simulink model "linear_pto_example"  (R2014a)
settings: Solver=ode45  StartTime=0.0  StopTime=10.0  RelTol=1e-3
undefined symbols (not defined in the file or in its folder): A_bore, A_rod, body, Gen_Damp, hyd_mot_eff, Jtot, p_hp, pto, V_hp, V_tot, Vg
libraries: WECSim_Lib x3
settings Model: Creator=kmruehl  LastModifiedBy=kmruehl
settings DebuggingCC: UnderspecifiedInitializationDetection=Classic  StateNameClashWarn=warning

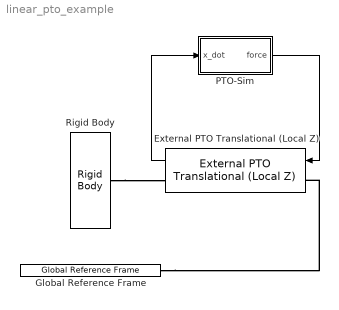
== system linear_pto_example ==
  External PTO Translational (Local Z) : WECSim_Lib/PTOs/External PTO  Translational (Local Z)  pto=pto(1)
      settings: AttributesFormatString=%<pto>
  Global Reference Frame : WECSim_Lib/Frames/Global Reference Frame  waves=waves  simu=simu
  PTO-Sim : Subsystem
  Rigid Body : WECSim_Lib/Body Elements/Rigid Body  Coupling=No  body=body(1)
      settings: AttributesFormatString=%<body>
  wires:
  External PTO Translational (Local Z)/1 -> PTO-Sim/1(x_dot)
  PTO-Sim/1(force) -> External PTO Translational (Local Z)/1
  connections:
  Rigid Body/RConn1 -- External PTO Translational (Local Z)/RConn1
  Global Reference Frame/RConn1 -- External PTO Translational (Local Z)/LConn1

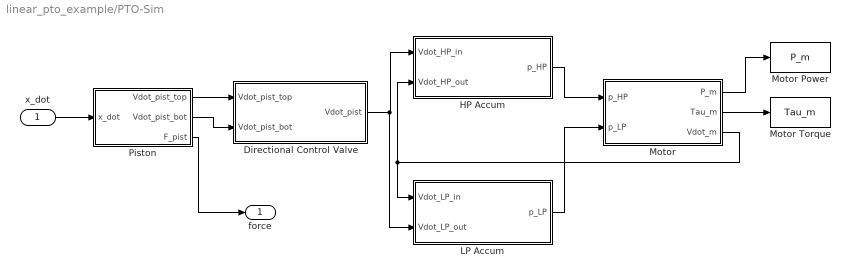
== system linear_pto_example/PTO-Sim ==
  x_dot : Inport
  Directional Control Valve : Subsystem
  HP Accum : Subsystem
  LP Accum : Subsystem
  Motor : Subsystem
  Motor Power : ToWorkspace  VariableName=P_m  SaveFormat=Timeseries  SampleTime=-1
  Motor Torque : ToWorkspace  VariableName=Tau_m  SaveFormat=Timeseries  SampleTime=-1
  Piston : Subsystem
  force : Outport
  wires:
  x_dot/1 -> Piston/1(x_dot)
  Motor/1(P_m) -> Motor Power/1
  Motor/2(Tau_m) -> Motor Torque/1
  Piston/2(Vdot_pist_bot) -> Directional Control Valve/2(Vdot_pist_bot)
  Piston/1(Vdot_pist_top) -> Directional Control Valve/1(Vdot_pist_top)
  Directional Control Valve/1(Vdot_pist) -> LP Accum/2(Vdot_LP_out), HP Accum/1(Vdot_HP_in)
  HP Accum/1(p_HP) -> Motor/1(p_HP)
  LP Accum/1(p_LP) -> Motor/2(p_LP)
  Motor/3(Vdot_m) -> LP Accum/1(Vdot_LP_in), HP Accum/2(Vdot_HP_out)
  Piston/3(F_pist) -> force/1

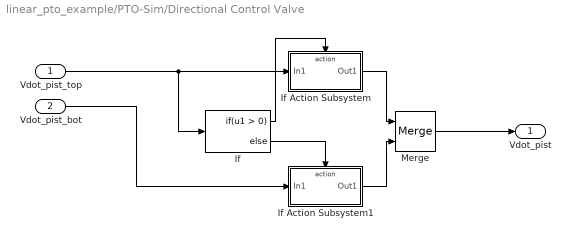
== system linear_pto_example/PTO-Sim/Directional Control Valve ==
  Vdot_pist_top : Inport
  Vdot_pist_bot : Inport  Port=2
  If : If
  If Action Subsystem : Subsystem  TreatAsAtomicUnit=on
  If Action Subsystem1 : Subsystem  TreatAsAtomicUnit=on
  Merge : Merge
  Vdot_pist : Outport
  wires:
  Vdot_pist_top/1 -> If/1, If Action Subsystem/1(In1)
  If/1 -> If Action Subsystem/Action
  If/2 -> If Action Subsystem1/Action
  If Action Subsystem/1(Out1) -> Merge/1
  If Action Subsystem1/1(Out1) -> Merge/2
  Vdot_pist_bot/1 -> If Action Subsystem1/1(In1)
  Merge/1 -> Vdot_pist/1

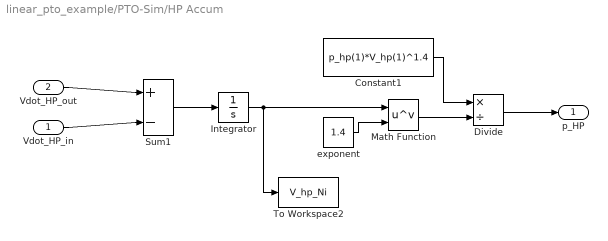
== system linear_pto_example/PTO-Sim/HP Accum ==
  Vdot_HP_in : Inport
  Vdot_HP_out : Inport  Port=2
  Constant1 : Constant  Value=p_hp(1)*V_hp(1)^1.4
  Divide : Product  Inputs=*/
  Integrator : Integrator  InitialCondition=V_hp(1)
  Math Function : Math  Operator=pow  SaturateOnIntegerOverflow=on
  Sum1 : Sum  Inputs=+|-
  To Workspace2 : ToWorkspace  VariableName=V_hp_Ni  SampleTime=-1
  exponent : Constant  Value=1.4
  p_HP : Outport
  wires:
  Integrator/1 -> Math Function/1, To Workspace2/1
  Divide/1 -> p_HP/1
  Math Function/1 -> Divide/2
  exponent/1 -> Math Function/2
  Constant1/1 -> Divide/1
  Sum1/1 -> Integrator/1
  Vdot_HP_in/1 -> Sum1/2
  Vdot_HP_out/1 -> Sum1/1

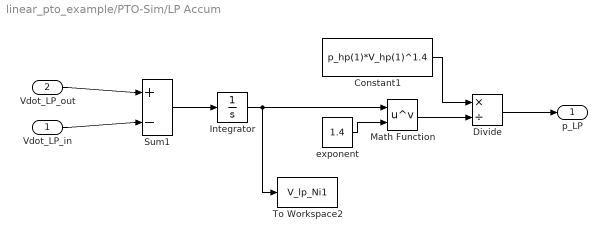
== system linear_pto_example/PTO-Sim/LP Accum ==
  Vdot_LP_in : Inport
  Vdot_LP_out : Inport  Port=2
  Constant1 : Constant  Value=p_hp(1)*V_hp(1)^1.4
  Divide : Product  Inputs=*/
  Integrator : Integrator  InitialCondition=V_hp(1)
  Math Function : Math  Operator=pow  SaturateOnIntegerOverflow=on
  Sum1 : Sum  Inputs=+|-
  To Workspace2 : ToWorkspace  VariableName=V_lp_Ni1  SampleTime=-1
  exponent : Constant  Value=1.4
  p_LP : Outport
  wires:
  Integrator/1 -> Math Function/1, To Workspace2/1
  Divide/1 -> p_LP/1
  Math Function/1 -> Divide/2
  exponent/1 -> Math Function/2
  Constant1/1 -> Divide/1
  Sum1/1 -> Integrator/1
  Vdot_LP_in/1 -> Sum1/2
  Vdot_LP_out/1 -> Sum1/1

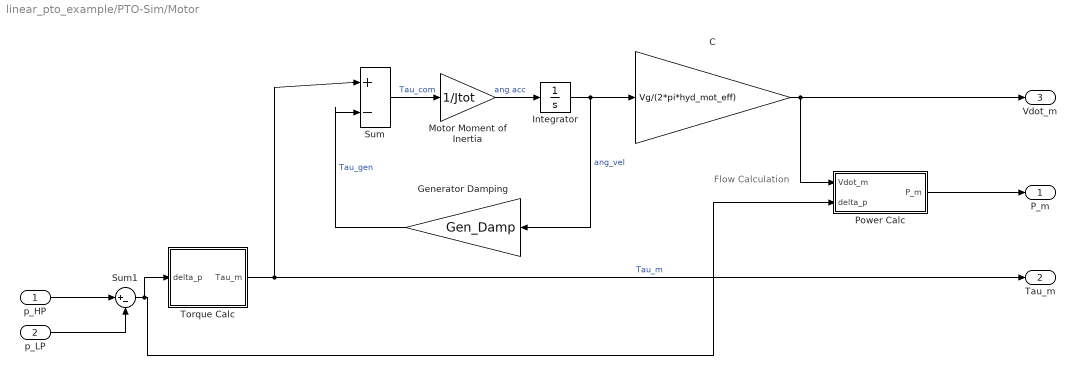
== system linear_pto_example/PTO-Sim/Motor ==
  note: Flow
      | Calculation
  p_HP : Inport
  p_LP : Inport  Port=2
  C : Gain  Gain=Vg/(2*pi*hyd_mot_eff)
  Generator Damping : Gain  Gain=Gen_Damp
  Integrator : Integrator
  Motor Moment of Inertia : Gain  Gain=1/Jtot
  Power Calc : Subsystem
  Sum : Sum  Inputs=|+|-|
  Sum1 : Sum  Inputs=|+-
  Torque Calc : Subsystem
  P_m : Outport
  Tau_m : Outport  Port=2
  Vdot_m : Outport  Port=3
  wires:
  Power Calc/1(P_m) -> P_m/1
  Sum/1 -> Motor Moment of Inertia/1  "Tau_com"
  Motor Moment of Inertia/1 -> Integrator/1  "ang acc"
  Integrator/1 -> Generator Damping/1, C/1  "ang_vel"
  Torque Calc/1(Tau_m) -> Sum/1, Tau_m/1  "Tau_m"
  Generator Damping/1 -> Sum/2  "Tau_gen"
  C/1 -> Power Calc/1(Vdot_m), Vdot_m/1
  p_HP/1 -> Sum1/1
  p_LP/1 -> Sum1/2
  Sum1/1 -> Torque Calc/1(delta_p), Power Calc/2(delta_p)

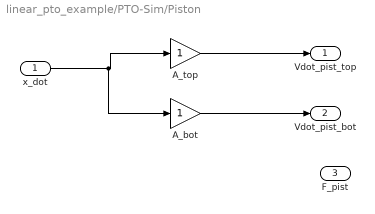
== system linear_pto_example/PTO-Sim/Piston ==
  x_dot : Inport
  A_bot : Gain
  A_top : Gain
  Vdot_pist_top : Outport
  Vdot_pist_bot : Outport  Port=2
  F_pist : Outport  Port=3
  wires:
  x_dot/1 -> A_bot/1, A_top/1
  A_top/1 -> Vdot_pist_top/1
  A_bot/1 -> Vdot_pist_bot/1

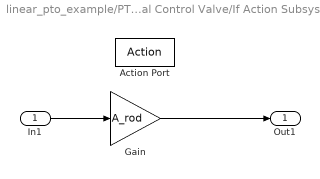
== system linear_pto_example/PTO-Sim/Directional Control Valve/If Action Subsystem ==
  In1 : Inport
  Action Port : ActionPort
  Gain : Gain  Gain=A_rod
  Out1 : Outport
  wires:
  In1/1 -> Gain/1
  Gain/1 -> Out1/1

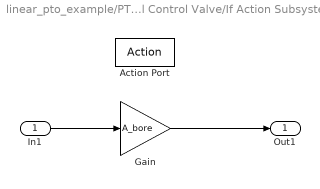
== system linear_pto_example/PTO-Sim/Directional Control Valve/If Action Subsystem1 ==
  In1 : Inport
  Action Port : ActionPort
  Gain : Gain  Gain=A_bore
  Out1 : Outport
  wires:
  In1/1 -> Gain/1
  Gain/1 -> Out1/1

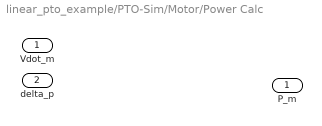
== system linear_pto_example/PTO-Sim/Motor/Power Calc ==
  Vdot_m : Inport
  delta_p : Inport  Port=2
  P_m : Outport

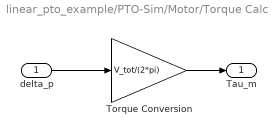
== system linear_pto_example/PTO-Sim/Motor/Torque Calc ==
  delta_p : Inport
  Torque Conversion : Gain  Gain=V_tot/(2*pi)
  Tau_m : Outport
  wires:
  Torque Conversion/1 -> Tau_m/1
  delta_p/1 -> Torque Conversion/1
